simulink model "Australian14gen_R2017a"  (R2017a)
settings: Solver=ode23tb  StartTime=0.0  StopTime=50  FixedStep=1/50  MaxStep=1/50  RelTol=1e-3  AbsTol=1e-1  EnableMultiTasking=on
PreLoadFcn:
  | dataaustralian14gen
values from neighbouring files (symbols this model uses):
  bus_v = [ 101	15 ... (first row only)    [dataaustralian14gen.m]
  comp = [ 1	211	0	0 ... (first row only)    [dataaustralian14gen.m]
  Exc = [ 101	0	 200	0.1	    13.25  2.5	 0	0       0       0       0       0 ... (first row only)    [dataaustralian14gen.m]
  FH = 13    [dataaustralian14gen.m]
  FI = 1    [dataaustralian14gen.m]
  FL = .1    (= 0.1)    [dataaustralian14gen.m]
  G_data = [ 101	333.3	15	3.6	0.14	1.1	0.65	0.25	8.5     0.20	0.05	0       0       0.25	0.2 	0 ... (first row only)    [dataaustralian14gen.m]
  KH = 120    [dataaustralian14gen.m]
  KI = 10    [dataaustralian14gen.m]
  KL = 10    [dataaustralian14gen.m]
  line = [ 102	217	0.0084	0.0667	0.817	330	1 ... (first row only)    [dataaustralian14gen.m]
  p = p_case1    [dataaustralian14gen.m]
  PSSMODEL = 1    [dataaustralian14gen.m]
  SVC = [ 205	650 430   -220 1.055  -68.3 ... (first row only)    [dataaustralian14gen.m]
  trans = [     1   101   102    15   330   333.3    12     12    0.9390 ... (first row only)    [dataaustralian14gen.m]
undefined symbols (not defined in the file or in its folder): D1, Delta
libraries: powerlib x371, sps_avr x14, powerlib_extras x9, factslib x5
(part 3 of 3)

== system Australian14gen_R2017a/NPS_5 ==
  501 : powerlib/Machines/Synchronous Machine pu Standard  PresetModel=No  MechanicalLoad=Mechanical power Pm  ShowDetailedParameters=on  RotorType=Round  Units=per unit standard parameters  MeasurementBus=off  NominalParameters="[G_data(12,2)*1E6  G_data(12,3)*1E3  50]"  Reactances1=[G_data(12,6),G_data(12,8),G_data(12,10),G_data(12,7),G_data(12,12),G_data(12,14),G_data(12,5)]  Reactances2=[G_data(12,6),G_data(12,8),G_data(12,10),G_data(12,7),G_data(12,12),G_data(12,14),G_data(12,5)]  dAxisTimeConstants=Open-circuit  qAxisTimeConstants=Open-circuit  TimeConstants1="[G_data(12,9)  G_data(12,11)  G_data(12,13) G_data(12,15)]"  TimeConstants2="[G_data(12,9)  G_data(12,11)  G_data(12,13) G_data(12,15)]"  TimeConstants3="[  5.9  0.033  0.023  ]"  TimeConstants4=[ 8.0, 0.03, 0.3371, 0.0295 ]  TimeConstants5=[ 1.01, 0.053, 0.1 ]  TimeConstants6=[ 1.3201, 0.023, 1.0, 0.07 ]  TimeConstants7="[  1.01  0.053  0.051266  ]"  TimeConstants8=[ 1.3201, 0.0231, 0.3371, 0.0295 ]  StatorResistance=0  Mechanical="[ G_data(12,4) 0  4 ]"  PolePairs=4  InitialConditions=[0 -93.632 0.904595 0.904595 0.904595 -62.347 -182.347 57.653 2.30263]  SetSaturation=off  Saturation=[0.6404,0.7127,0.8441,0.9214,0.9956,1.082,1.19,1.316,1.457;0.7,0.7698,0.8872,0.9466,0.9969,1.046,1.1,1.151,1.201]  LoadFlowParameters=[1 600000000 20000 0 0]  TsPowergui=0  TsBlock=-1  IterativeModel=Forward Euler  IterativeDiscreteModel=Trapezoidal non iterative  BusType=PV  Pref=p(12,3)*1e6  Qref=0  Qmin=-inf  Qmax=inf  PLF=0  QLF=0
      settings: SourceProductName=Simscape Power Systems
  AC1A Excitation System 501 : sps_avr/AC1A Excitation System  Tr=Exc(12,2)  KaTa="[Exc(12,3)   Exc(12,4)]"  VAminmax=[-14.5 14.5]  VRminmax=[-5.43 6.03]  KfTf="[Exc(12,9)  Exc(12,10)]"  TbTc="[Exc(12,5)  Exc(12,6)]"  KeTe="[Exc(12,7)  Exc(12,8)]"  Ve12=[4.18 3.14]  SeVe12=[0.10 0.03]  Kd=0.38  Kc=0.20  v0=[1 2.3026]  TsBlock=0
      settings: SourceProductName=Simscape Power Systems  SourceProductBaseCode=PS
  Bus Selector1 : BusSelector  OutputSignals="Mechanical.Rotor speed  wm  (pu),Output active power   Peo (pu),Mechanical.Rotor speed deviation  dw (pu),Mechanical.Rotor angle deviation  d_theta (rad),Mechanical.Rotor mechanical angle  theta (deg),dq0 components.Stator voltage  vd (pu),dq0 components.Stator voltage  vq (pu),dq0 components.Field current  ifd (pu),Output reactive power  Qeo (pu)"
  Complex to Magnitude-Angle : ComplexToMagnitudeAngle  Output=Magnitude
  "Delta Pa PSS 501 " : powerlib/Machines/Generic Power System Stabilizer  Tsensor=15e-3  K=2.5*1.25  Twashout=1  Tleadlag1=[60e-3 1]  Tleadlag2=[0 0]  VSlimits=[-0.15 0.15]  Vinit=0  Plot_On=off  MagdB_On=on  FreqRange=logspace(-2,2,500)
      settings: SourceProductName=Simscape Power Systems  SourceProductBaseCode=PS
  "Delta w PSS (Kundur) 501 " : powerlib/Machines/Generic Power System Stabilizer  Tsensor=15e-3  K=30  Twashout=10  Tleadlag1=[50e-3 20e-3]  Tleadlag2=[3 5.4]  VSlimits=[-0.15 0.15]  Vinit=0  Plot_On=off  MagdB_On=on  FreqRange=logspace(-2,2,500)
      settings: SourceProductName=Simscape Power Systems  SourceProductBaseCode=PS
  "MB-PSS 501 " : powerlib/Machines/Multi-Band Power System Stabilizer  OperationMode=Simplified settings  Kg=G  GL="[FL  KL]"  GI="[FI  KI]"  GH="[FH  KH]"  GLd=[66 66 9.4]  TcLF=[1.667 2 0 0 0 0 2 2.4 0 0 0 0 1 1]  GId=[66 66 47.6]  TcIF=[1 1 0.25 0.3 0 0 1 1 0.3 0.36 0 0 0 0]  GHd=[66 66 233]  TcHF="[0.01 0.012 0 0 0 0  0.012 0.0144 0 0 0 0 1 1]"  LIM=[.075 .15 .15 .15]  Plot_On=off  MagdB_On=off  FreqRange=logspace(-2,2,500)
      settings: SourceProductName=Simscape Power Systems  SourceProductBaseCode=PS
  Multiport Switch1 : MultiPortSwitch  Inputs=4  InputSameDT=on
  PSS model3 : Constant  Value=0
  PSS model4 : Constant
  Pref1 : Constant  Value=0.90009
  Real-Imag to Complex : RealImagToComplex
  STG 501 : powerlib/Machines/Steam Turbine and Governor  gentype=Tandem-compound (single mass)  reg1="[ 1  0.05    0 ]"  reg2="[ 0.001  0.15 ]"  reg3="[ -0.1  0.1  0  4.496 ]"  N=3000  turb1="[ 0  10   3.3   0.5   ]"  turb2="[   0   0.36    0.36   0.28   ]"  HA="[ 0.046  1.430  1.465   0.192 ]"  KA="[ 90.44  53.88  64.59   62.94  ]"  DA="[ 0.0115  0.3575  0.3663   0.0137  ]"  ini1=0.90009  ini2=[0.779316,-31.4247]
      settings: SourceProductName=Simscape Power Systems  SourceProductBaseCode=PS
  Scope4 : Scope
  Sum2 : Sum  SaturateOnIntegerOverflow=on  InputSameDT=on  OutDataTypeStr=Inherit: Same as first input
  Sum3 : Sum  Inputs=-+  SaturateOnIntegerOverflow=on  InputSameDT=on  OutDataTypeStr=Inherit: Same as first input
  Vref501 : Constant
  wref : Constant
  A : PMIOPort  Port=1  Side=Left
  B : PMIOPort  Port=2  Side=Left
  C : PMIOPort  Port=3  Side=Left
  tag scope: EFD501=global, Pa501=global, Pe501=global, Pm501=global, Q501=global, Vt501=global, d_theta501=global, pss501=global, theta501=global, w501=global
  wires:
  Bus Selector1/7 -> Real-Imag to Complex/2  "<Stator voltage  vq (pu)>"
  Bus Selector1/6 -> Real-Imag to Complex/1  "<Stator voltage  vd (pu)>"
  wref/1 -> STG 501/1
  Vref501/1 -> AC1A Excitation System 501/1
  Bus Selector1/4 -> STG 501/4, [d_theta501]  "<Rotor angle deviation  d_theta (rad)>"
  501/1 -> [M501], Bus Selector1/1
  Bus Selector1/1 -> [w501], STG 501/3  "<Rotor speed  wm  (pu)>"
  Bus Selector1/3 -> "Delta w PSS (Kundur) 501 "/1, "MB-PSS 501 "/1  "<Rotor speed deviation  dw (pu)>"
  Real-Imag to Complex/1 -> Complex to Magnitude-Angle/1
  Complex to Magnitude-Angle/1 -> AC1A Excitation System 501/2, [Vt501]
  AC1A Excitation System 501/1 -> 501/2, [EFD501]
  Bus Selector1/5 -> [theta501]  "<Rotor mechanical angle  theta (deg)>"
  Bus Selector1/2 -> [Pe501]  "<Output active power   Peo (pu)>"
  Bus Selector1/8 -> AC1A Excitation System 501/3  "<Field current  ifd (pu)>"
  STG 501/4 -> 501/1, [Pm501]
  Bus Selector1/9 -> [Q501]  "<Output reactive power  Qeo (pu)>"
  PSS model4/1 -> Sum2/2
  Sum2/1 -> Multiport Switch1/1
  [PSSmodel] -> Sum2/1
  PSS model3/1 -> Multiport Switch1/2
  Sum3/1 -> [Pa501], "Delta Pa PSS 501 "/1  "Pm-Pe"
  "Delta Pa PSS 501 "/1 -> Multiport Switch1/5
  "Delta w PSS (Kundur) 501 "/1 -> Multiport Switch1/4
  [Pm501] -> Sum3/2
  [Pe501] -> Sum3/1
  "MB-PSS 501 "/1 -> Multiport Switch1/3
  Pref1/1 -> STG 501/2
  Multiport Switch1/1 -> AC1A Excitation System 501/4, Scope4/1, [pss501]
  connections:
  501/RConn1 -- A/RConn1
  501/RConn2 -- B/RConn1
  501/RConn3 -- C/RConn1

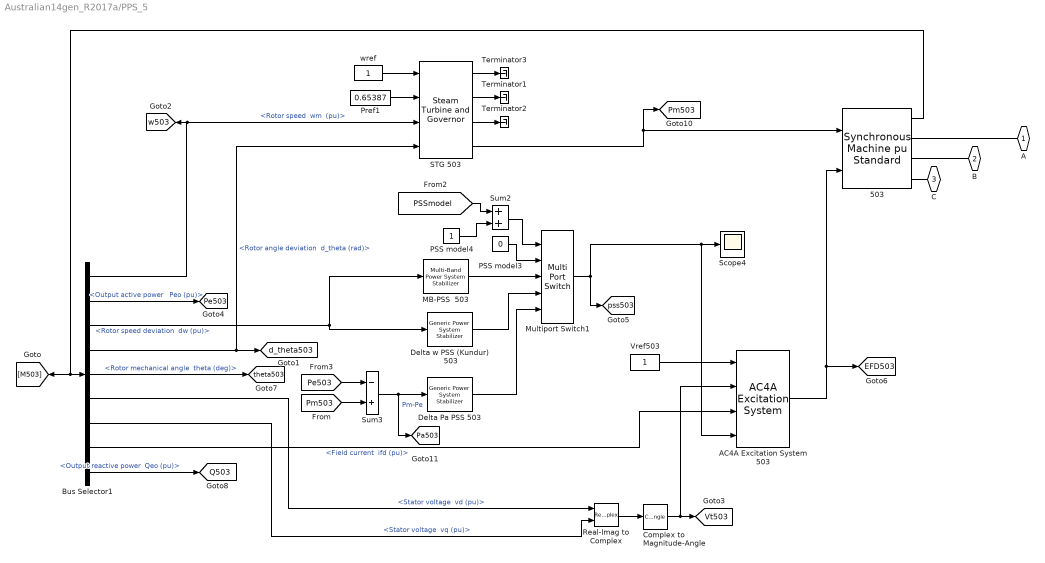
== system Australian14gen_R2017a/PPS_5 ==
  503 : powerlib/Machines/Synchronous Machine pu Standard  PresetModel=No  MechanicalLoad=Mechanical power Pm  ShowDetailedParameters=on  RotorType=Round  Units=per unit standard parameters  MeasurementBus=off  NominalParameters="[G_data(14,2)*1E6  G_data(14,3)*1E3  50]"  Reactances1=[G_data(14,6),G_data(14,8),G_data(14,10),G_data(14,7),G_data(14,12),G_data(14,14),G_data(14,5)]  Reactances2=[G_data(14,6),G_data(14,8),G_data(14,10),G_data(14,7),G_data(14,12),G_data(14,14),G_data(14,5)]  dAxisTimeConstants=Open-circuit  qAxisTimeConstants=Open-circuit  TimeConstants1="[G_data(14,9)  G_data(14,11) G_data(14,13)  G_data(14,15)]"  TimeConstants2="[G_data(14,9)  G_data(14,11) G_data(14,13)  G_data(14,15)]"  TimeConstants3="[  5.9  0.033  0.023  ]"  TimeConstants4=[ 8.0, 0.03, 0.3371, 0.0295 ]  TimeConstants5=[ 1.01, 0.053, 0.1 ]  TimeConstants6=[ 1.3201, 0.023, 1.0, 0.07 ]  TimeConstants7="[  1.01  0.053  0.051266  ]"  TimeConstants8=[ 1.3201, 0.0231, 0.3371, 0.0295 ]  StatorResistance=0  Mechanical=[ G_data(14,4) 0 4 ]  PolePairs=4  InitialConditions=[0 -103.108 0.674862 0.674862 0.674862 -71.8664 -191.866 48.1336 2.0412]  SetSaturation=off  Saturation=[0.6404,0.7127,0.8441,0.9214,0.9956,1.082,1.19,1.316,1.457;0.7,0.7698,0.8872,0.9466,0.9969,1.046,1.1,1.151,1.201]  LoadFlowParameters=[1 436000000 15000 0 0]  TsPowergui=0  TsBlock=-1  IterativeModel=Forward Euler  IterativeDiscreteModel=Trapezoidal non iterative  BusType=PV  Pref=p(14,3)*1e6  Qref=0  Qmin=-inf  Qmax=inf  PLF=0  QLF=0
      settings: SourceProductName=Simscape Power Systems
  AC4A Excitation System 503 : sps_avr/AC4A Excitation System  Tr=Exc(14,2)  KaTa="[Exc(14,3)   Exc(14,4)]"  VIminmax=[-10 10]  VRminmax=[-4.53 5.64]  TbTc="[Exc(14,5)  Exc(14,6)]"  Kc=0  v0=[1 2.0412]  TsBlock=0
      settings: SourceProductName=Simscape Power Systems  SourceProductBaseCode=PS
  Bus Selector1 : BusSelector  OutputSignals="Mechanical.Rotor speed  wm  (pu),Output active power   Peo (pu),Mechanical.Rotor speed deviation  dw (pu),Mechanical.Rotor angle deviation  d_theta (rad),Mechanical.Rotor mechanical angle  theta (deg),dq0 components.Stator voltage  vd (pu),dq0 components.Stator voltage  vq (pu),dq0 components.Field current  ifd (pu),Output reactive power  Qeo (pu)"
  Complex to Magnitude-Angle : ComplexToMagnitudeAngle  Output=Magnitude
  "Delta Pa PSS 503 " : powerlib/Machines/Generic Power System Stabilizer  Tsensor=15e-3  K=2.5*1.25  Twashout=1  Tleadlag1=[60e-3 1]  Tleadlag2=[0 0]  VSlimits=[-0.15 0.15]  Vinit=0  Plot_On=off  MagdB_On=on  FreqRange=logspace(-2,2,500)
      settings: SourceProductName=Simscape Power Systems  SourceProductBaseCode=PS
  Delta w PSS (Kundur)  503 : powerlib/Machines/Generic Power System Stabilizer  Tsensor=15e-3  K=30  Twashout=10  Tleadlag1=[50e-3 20e-3]  Tleadlag2=[3 5.4]  VSlimits=[-0.15 0.15]  Vinit=0  Plot_On=off  MagdB_On=on  FreqRange=logspace(-2,2,500)
      settings: SourceProductName=Simscape Power Systems  SourceProductBaseCode=PS
  MB-PSS  503 : powerlib/Machines/Multi-Band Power System Stabilizer  OperationMode=Simplified settings  Kg=G  GL="[FL  KL]"  GI="[FI  KI]"  GH="[FH  KH]"  GLd=[66 66 9.4]  TcLF=[1.667 2 0 0 0 0 2 2.4 0 0 0 0 1 1]  GId=[66 66 47.6]  TcIF=[1 1 0.25 0.3 0 0 1 1 0.3 0.36 0 0 0 0]  GHd=[66 66 233]  TcHF="[0.01 0.012 0 0 0 0  0.012 0.0144 0 0 0 0 1 1]"  LIM=[.075 .15 .15 .15]  Plot_On=off  MagdB_On=off  FreqRange=logspace(-2,2,500)
      settings: SourceProductName=Simscape Power Systems  SourceProductBaseCode=PS
  Multiport Switch1 : MultiPortSwitch  Inputs=4  InputSameDT=on
  PSS model3 : Constant  Value=0
  PSS model4 : Constant
  Pref1 : Constant  Value=0.65387
  Real-Imag to Complex : RealImagToComplex
  STG 503 : powerlib/Machines/Steam Turbine and Governor  gentype=Tandem-compound (single mass)  reg1="[ 1  0.05    0 ]"  reg2="[ 0.001  0.15 ]"  reg3="[ -0.1  0.1  0  4.496 ]"  N=3000  turb1="[ 0  10   3.3   0.5   ]"  turb2="[   0   0.36    0.36   0.28   ]"  HA="[ 0.046  1.430  1.465   0.192 ]"  KA="[ 90.44  53.88  64.59   62.94  ]"  DA="[ 0.0115  0.3575  0.3663   0.0137  ]"  ini1=0.65387  ini2=[0.779316,-31.4247]
      settings: SourceProductName=Simscape Power Systems  SourceProductBaseCode=PS
  Scope4 : Scope
  Sum2 : Sum  SaturateOnIntegerOverflow=on  InputSameDT=on  OutDataTypeStr=Inherit: Same as first input
  Sum3 : Sum  Inputs=-+  SaturateOnIntegerOverflow=on  InputSameDT=on  OutDataTypeStr=Inherit: Same as first input
  Terminator1 : Terminator
  Terminator2 : Terminator
  Terminator3 : Terminator
  Vref503 : Constant
  wref : Constant
  A : PMIOPort  Port=1  Side=Left
  B : PMIOPort  Port=2  Side=Left
  C : PMIOPort  Port=3  Side=Left
  tag scope: EFD503=global, Pa503=global, Pe503=global, Pm503=global, Q503=global, Vt503=global, d_theta503=global, pss503=global, theta503=global, w503=global
  wires:
  Bus Selector1/7 -> Real-Imag to Complex/2  "<Stator voltage  vq (pu)>"
  Bus Selector1/6 -> Real-Imag to Complex/1  "<Stator voltage  vd (pu)>"
  wref/1 -> STG 503/1
  Vref503/1 -> AC4A Excitation System 503/1
  Bus Selector1/4 -> STG 503/4, [d_theta503]  "<Rotor angle deviation  d_theta (rad)>"
  503/1 -> [M503], Bus Selector1/1
  Bus Selector1/1 -> [w503], STG 503/3  "<Rotor speed  wm  (pu)>"
  Bus Selector1/3 -> MB-PSS  503/1, Delta w PSS (Kundur)  503/1  "<Rotor speed deviation  dw (pu)>"
  Real-Imag to Complex/1 -> Complex to Magnitude-Angle/1
  Complex to Magnitude-Angle/1 -> AC4A Excitation System 503/2, [Vt503]
  AC4A Excitation System 503/1 -> 503/2, [EFD503]
  Bus Selector1/5 -> [theta503]  "<Rotor mechanical angle  theta (deg)>"
  Bus Selector1/2 -> [Pe503]  "<Output active power   Peo (pu)>"
  Bus Selector1/8 -> AC4A Excitation System 503/3  "<Field current  ifd (pu)>"
  STG 503/4 -> 503/1, [Pm503]
  Bus Selector1/9 -> [Q503]  "<Output reactive power  Qeo (pu)>"
  PSS model4/1 -> Sum2/2
  Sum2/1 -> Multiport Switch1/1
  [PSSmodel] -> Sum2/1
  PSS model3/1 -> Multiport Switch1/2
  Sum3/1 -> [Pa503], "Delta Pa PSS 503 "/1  "Pm-Pe"
  "Delta Pa PSS 503 "/1 -> Multiport Switch1/5
  Delta w PSS (Kundur)  503/1 -> Multiport Switch1/4
  [Pm503] -> Sum3/2
  [Pe503] -> Sum3/1
  MB-PSS  503/1 -> Multiport Switch1/3
  STG 503/1 -> Terminator3/1
  STG 503/2 -> Terminator1/1
  STG 503/3 -> Terminator2/1
  Pref1/1 -> STG 503/2
  Multiport Switch1/1 -> AC4A Excitation System 503/4, Scope4/1, [pss503]
  connections:
  503/RConn1 -- A/RConn1
  503/RConn2 -- B/RConn1
  503/RConn3 -- C/RConn1

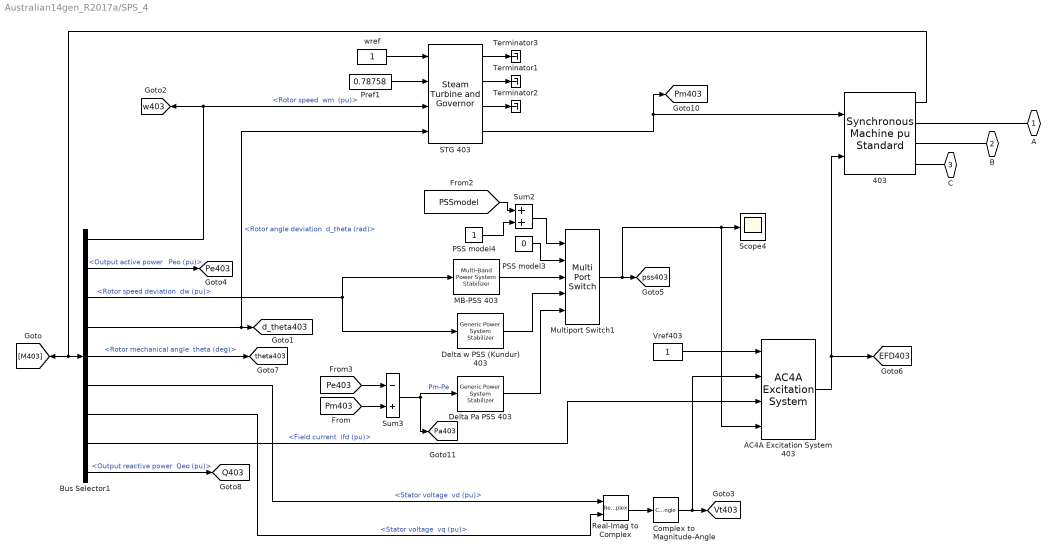
== system Australian14gen_R2017a/SPS_4 ==
  403 : powerlib/Machines/Synchronous Machine pu Standard  PresetModel=No  MechanicalLoad=Mechanical power Pm  ShowDetailedParameters=on  RotorType=Round  Units=per unit standard parameters  MeasurementBus=off  NominalParameters="[G_data(10,2)*1E6  G_data(10,3)*1E3  50]"  Reactances1=[G_data(10,6),G_data(10,8),G_data(10,10),G_data(10,7),G_data(10,12),G_data(10,14),G_data(10,5)]  Reactances2=[G_data(10,6),G_data(10,8),G_data(10,10),G_data(10,7),G_data(10,12),G_data(10,14),G_data(10,5)]  dAxisTimeConstants=Open-circuit  qAxisTimeConstants=Open-circuit  TimeConstants1="[G_data(10,9)  G_data(10,11)  G_data(10,13)  G_data(10,15)]"  TimeConstants2="[G_data(10,9)  G_data(10,11)  G_data(10,13)  G_data(10,15)]"  TimeConstants3="[  5.9  0.033  0.023  ]"  TimeConstants4=[ 8.0, 0.03, 0.3371, 0.0295 ]  TimeConstants5=[ 1.01, 0.053, 0.1 ]  TimeConstants6=[ 1.3201, 0.023, 1.0, 0.07 ]  TimeConstants7="[  1.01  0.053  0.051266  ]"  TimeConstants8=[ 1.3201, 0.0231, 0.3371, 0.0295 ]  StatorResistance=0  Mechanical="[ G_data(10,4) 0  4 ]"  PolePairs=4  InitialConditions=[0 67.1142 0.796278 0.796278 0.796278 100.495 -19.5047 220.495 2.1966]  SetSaturation=off  Saturation=[0.6404,0.7127,0.8441,0.9214,0.9956,1.082,1.19,1.316,1.457;0.7,0.7698,0.8872,0.9466,0.9969,1.046,1.1,1.151,1.201]  LoadFlowParameters=[1 1400000000 20000 0 0]  TsPowergui=0  TsBlock=-1  IterativeModel=Forward Euler  IterativeDiscreteModel=Trapezoidal non iterative  BusType=PV  Pref=p(10,3)*1e6  Qref=0  Qmin=-inf  Qmax=inf  PLF=0  QLF=0
      settings: SourceProductName=Simscape Power Systems
  AC4A Excitation System 403 : sps_avr/AC4A Excitation System  Tr=Exc(10,2)  KaTa="[Exc(10,3)   Exc(10,4)]"  VIminmax=[-10 10]  VRminmax=[-4.53 5.64]  TbTc="[Exc(10,5)  Exc(10,6)]"  Kc=0  v0=[1 2.1966]  TsBlock=0
      settings: SourceProductName=Simscape Power Systems  SourceProductBaseCode=PS
  Bus Selector1 : BusSelector  OutputSignals="Mechanical.Rotor speed  wm  (pu),Output active power   Peo (pu),Mechanical.Rotor speed deviation  dw (pu),Mechanical.Rotor angle deviation  d_theta (rad),Mechanical.Rotor mechanical angle  theta (deg),dq0 components.Stator voltage  vd (pu),dq0 components.Stator voltage  vq (pu),dq0 components.Field current  ifd (pu),Output reactive power  Qeo (pu)"
  Complex to Magnitude-Angle : ComplexToMagnitudeAngle  Output=Magnitude
  "Delta Pa PSS 403 " : powerlib/Machines/Generic Power System Stabilizer  Tsensor=15e-3  K=2.5*1.25  Twashout=1  Tleadlag1=[60e-3 1]  Tleadlag2=[0 0]  VSlimits=[-0.15 0.15]  Vinit=0  Plot_On=off  MagdB_On=on  FreqRange=logspace(-2,2,500)
      settings: SourceProductName=Simscape Power Systems  SourceProductBaseCode=PS
  Delta w PSS (Kundur) 403 : powerlib/Machines/Generic Power System Stabilizer  Tsensor=15e-3  K=30  Twashout=10  Tleadlag1=[50e-3 20e-3]  Tleadlag2=[3 5.4]  VSlimits=[-0.15 0.15]  Vinit=0  Plot_On=off  MagdB_On=on  FreqRange=logspace(-2,2,500)
      settings: SourceProductName=Simscape Power Systems  SourceProductBaseCode=PS
  "MB-PSS 403 " : powerlib/Machines/Multi-Band Power System Stabilizer  OperationMode=Simplified settings  Kg=G  GL="[FL  KL]"  GI="[FI  KI]"  GH="[FH  KH]"  GLd=[66 66 9.4]  TcLF=[1.667 2 0 0 0 0 2 2.4 0 0 0 0 1 1]  GId=[66 66 47.6]  TcIF=[1 1 0.25 0.3 0 0 1 1 0.3 0.36 0 0 0 0]  GHd=[66 66 233]  TcHF="[0.01 0.012 0 0 0 0  0.012 0.0144 0 0 0 0 1 1]"  LIM=[.075 .15 .15 .15]  Plot_On=off  MagdB_On=off  FreqRange=logspace(-2,2,500)
      settings: SourceProductName=Simscape Power Systems  SourceProductBaseCode=PS
  Multiport Switch1 : MultiPortSwitch  Inputs=4  InputSameDT=on
  PSS model3 : Constant  Value=0
  PSS model4 : Constant
  Pref1 : Constant  Value=0.78758
  Real-Imag to Complex : RealImagToComplex
  STG 403 : powerlib/Machines/Steam Turbine and Governor  gentype=Tandem-compound (single mass)  reg1="[ 1  0.05    0 ]"  reg2="[ 0.001  0.15 ]"  reg3="[ -0.1  0.1  0  4.496 ]"  N=3000  turb1="[ 0  10   3.3   0.5   ]"  turb2="[   0   0.36    0.36   0.28   ]"  HA="[ 0.046  1.430  1.465   0.192 ]"  KA="[ 90.44  53.88  64.59   62.94  ]"  DA="[ 0.0115  0.3575  0.3663   0.0137  ]"  ini1=0.78758  ini2=[0.779316,-31.4247]
      settings: SourceProductName=Simscape Power Systems  SourceProductBaseCode=PS
  Scope4 : Scope
  Sum2 : Sum  SaturateOnIntegerOverflow=on  InputSameDT=on  OutDataTypeStr=Inherit: Same as first input
  Sum3 : Sum  Inputs=-+  SaturateOnIntegerOverflow=on  InputSameDT=on  OutDataTypeStr=Inherit: Same as first input
  Terminator1 : Terminator
  Terminator2 : Terminator
  Terminator3 : Terminator
  Vref403 : Constant
  wref : Constant
  A : PMIOPort  Port=1  Side=Left
  B : PMIOPort  Port=2  Side=Left
  C : PMIOPort  Port=3  Side=Left
  tag scope: EFD403=global, Pa403=global, Pe403=global, Pm403=global, Q403=global, Vt403=global, d_theta403=global, pss403=global, theta403=global, w403=global
  wires:
  Bus Selector1/7 -> Real-Imag to Complex/2  "<Stator voltage  vq (pu)>"
  Bus Selector1/6 -> Real-Imag to Complex/1  "<Stator voltage  vd (pu)>"
  wref/1 -> STG 403/1
  Vref403/1 -> AC4A Excitation System 403/1
  Bus Selector1/4 -> STG 403/4, [d_theta403]  "<Rotor angle deviation  d_theta (rad)>"
  403/1 -> [M403], Bus Selector1/1
  Bus Selector1/1 -> [w403], STG 403/3  "<Rotor speed  wm  (pu)>"
  Bus Selector1/3 -> Delta w PSS (Kundur) 403/1, "MB-PSS 403 "/1  "<Rotor speed deviation  dw (pu)>"
  Real-Imag to Complex/1 -> Complex to Magnitude-Angle/1
  Complex to Magnitude-Angle/1 -> AC4A Excitation System 403/2, [Vt403]
  AC4A Excitation System 403/1 -> 403/2, [EFD403]
  Bus Selector1/5 -> [theta403]  "<Rotor mechanical angle  theta (deg)>"
  Bus Selector1/2 -> [Pe403]  "<Output active power   Peo (pu)>"
  Bus Selector1/8 -> AC4A Excitation System 403/3  "<Field current  ifd (pu)>"
  STG 403/4 -> 403/1, [Pm403]
  Bus Selector1/9 -> [Q403]  "<Output reactive power  Qeo (pu)>"
  PSS model4/1 -> Sum2/2
  Sum2/1 -> Multiport Switch1/1
  [PSSmodel] -> Sum2/1
  PSS model3/1 -> Multiport Switch1/2
  Sum3/1 -> [Pa403], "Delta Pa PSS 403 "/1  "Pm-Pe"
  "Delta Pa PSS 403 "/1 -> Multiport Switch1/5
  Delta w PSS (Kundur) 403/1 -> Multiport Switch1/4
  [Pm403] -> Sum3/2
  [Pe403] -> Sum3/1
  "MB-PSS 403 "/1 -> Multiport Switch1/3
  STG 403/1 -> Terminator3/1
  STG 403/2 -> Terminator1/1
  STG 403/3 -> Terminator2/1
  Pref1/1 -> STG 403/2
  Multiport Switch1/1 -> AC4A Excitation System 403/4, Scope4/1, [pss403]
  connections:
  403/RConn1 -- A/RConn1
  403/RConn2 -- B/RConn1
  403/RConn3 -- C/RConn1

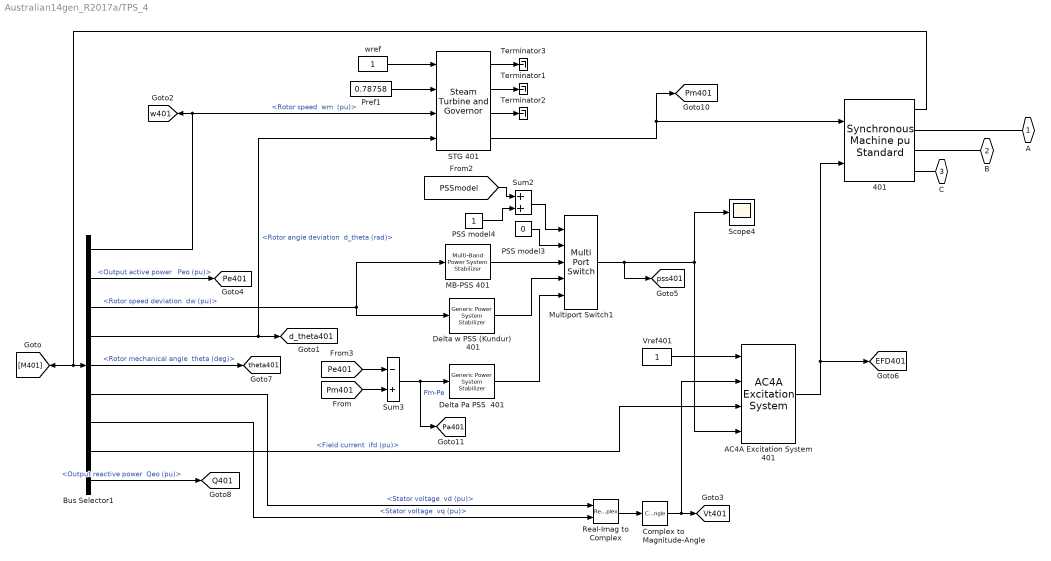
== system Australian14gen_R2017a/TPS_4 ==
  401 : powerlib/Machines/Synchronous Machine pu Standard  PresetModel=No  MechanicalLoad=Mechanical power Pm  ShowDetailedParameters=on  RotorType=Round  Units=per unit standard parameters  MeasurementBus=off  NominalParameters="[G_data(8,2)*1E6  G_data(8,3)*1E3  50]"  Reactances1=[G_data(8,6),G_data(8,8),G_data(8,10),G_data(8,7),G_data(8,12),G_data(8,14),G_data(8,5)]  Reactances2=[G_data(8,6),G_data(8,8),G_data(8,10),G_data(8,7),G_data(8,14),G_data(8,5)]  dAxisTimeConstants=Open-circuit  qAxisTimeConstants=Open-circuit  TimeConstants1="[G_data(8,9)  G_data(8,11)  G_data(8,15)]"  TimeConstants2="[G_data(8,9)  G_data(8,11)  G_data(8,13)  G_data(8,15)]"  TimeConstants3="[  5.9  0.033  0.023  ]"  TimeConstants4=[ 8.0, 0.03, 0.3371, 0.0295 ]  TimeConstants5=[ 1.01, 0.053, 0.1 ]  TimeConstants6=[ 1.3201, 0.023, 1.0, 0.07 ]  TimeConstants7="[  1.01  0.053  0.051266  ]"  TimeConstants8=[ 1.3201, 0.0231, 0.3371, 0.0295 ]  StatorResistance=0  Mechanical="[ G_data(8,4) 0  4 ]"  PolePairs=4  InitialConditions=[0 23.0374 0.837012 0.837012 0.837012 51.1473 -68.8527 171.147 2.44002]  SetSaturation=off  Saturation=[0.6404,0.7127,0.8441,0.9214,0.9956,1.082,1.19,1.316,1.457;0.7,0.7698,0.8872,0.9466,0.9969,1.046,1.1,1.151,1.201]  LoadFlowParameters=[1 1400000000 20000 0 0]  TsPowergui=0  TsBlock=-1  IterativeModel=Forward Euler  IterativeDiscreteModel=Trapezoidal non iterative  BusType=PV  Pref=p(8,3)*1e6  Qref=0  Qmin=-inf  Qmax=inf  PLF=0  QLF=0
      settings: SourceProductName=Simscape Power Systems
  AC4A Excitation System 401 : sps_avr/AC4A Excitation System  Tr=Exc(8,2)  KaTa="[Exc(8,3)   Exc(8,4)]"  VIminmax=[-10 10]  VRminmax=[-4.53 5.64]  TbTc="[Exc(8,5)  Exc(8,6)]"  Kc=0  v0=[1 2.44]  TsBlock=0
      settings: SourceProductName=Simscape Power Systems  SourceProductBaseCode=PS
  Bus Selector1 : BusSelector  OutputSignals="Mechanical.Rotor speed  wm  (pu),Output active power   Peo (pu),Mechanical.Rotor speed deviation  dw (pu),Mechanical.Rotor angle deviation  d_theta (rad),Mechanical.Rotor mechanical angle  theta (deg),dq0 components.Stator voltage  vd (pu),dq0 components.Stator voltage  vq (pu),dq0 components.Field current  ifd (pu),Output reactive power  Qeo (pu)"
  Complex to Magnitude-Angle : ComplexToMagnitudeAngle  Output=Magnitude
  Delta Pa PSS  401 : powerlib/Machines/Generic Power System Stabilizer  Tsensor=15e-3  K=2.5*1.25  Twashout=1  Tleadlag1=[60e-3 1]  Tleadlag2=[0 0]  VSlimits=[-0.15 0.15]  Vinit=0  Plot_On=off  MagdB_On=on  FreqRange=logspace(-2,2,500)
      settings: SourceProductName=Simscape Power Systems  SourceProductBaseCode=PS
  Delta w PSS (Kundur)  401 : powerlib/Machines/Generic Power System Stabilizer  Tsensor=15e-3  K=30  Twashout=10  Tleadlag1=[50e-3 20e-3]  Tleadlag2=[3 5.4]  VSlimits=[-0.15 0.15]  Vinit=0  Plot_On=off  MagdB_On=on  FreqRange=logspace(-2,2,500)
      settings: SourceProductName=Simscape Power Systems  SourceProductBaseCode=PS
  "MB-PSS 401 " : powerlib/Machines/Multi-Band Power System Stabilizer  OperationMode=Simplified settings  Kg=G  GL="[FL  KL]"  GI="[FI  KI]"  GH="[FH  KH]"  GLd=[66 66 9.4]  TcLF=[1.667 2 0 0 0 0 2 2.4 0 0 0 0 1 1]  GId=[66 66 47.6]  TcIF=[1 1 0.25 0.3 0 0 1 1 0.3 0.36 0 0 0 0]  GHd=[66 66 233]  TcHF="[0.01 0.012 0 0 0 0  0.012 0.0144 0 0 0 0 1 1]"  LIM=[.075 .15 .15 .15]  Plot_On=off  MagdB_On=off  FreqRange=logspace(-2,2,500)
      settings: SourceProductName=Simscape Power Systems  SourceProductBaseCode=PS
  Multiport Switch1 : MultiPortSwitch  Inputs=4  InputSameDT=on
  PSS model3 : Constant  Value=0
  PSS model4 : Constant
  Pref1 : Constant  Value=0.78758
  Real-Imag to Complex : RealImagToComplex
  STG 401 : powerlib/Machines/Steam Turbine and Governor  gentype=Tandem-compound (single mass)  reg1="[ 1  0.05    0 ]"  reg2="[ 0.001  0.15 ]"  reg3="[ -0.1  0.1  0  4.496 ]"  N=3000  turb1="[ 0  10   3.3   0.5   ]"  turb2="[   0   0.36    0.36   0.28   ]"  HA="[ 0.046  1.430  1.465   0.192 ]"  KA="[ 90.44  53.88  64.59   62.94  ]"  DA="[ 0.0115  0.3575  0.3663   0.0137  ]"  ini1=0.78758  ini2=[0.779316,-31.4247]
      settings: SourceProductName=Simscape Power Systems  SourceProductBaseCode=PS
  Scope4 : Scope
  Sum2 : Sum  SaturateOnIntegerOverflow=on  InputSameDT=on  OutDataTypeStr=Inherit: Same as first input
  Sum3 : Sum  Inputs=-+  SaturateOnIntegerOverflow=on  InputSameDT=on  OutDataTypeStr=Inherit: Same as first input
  Terminator1 : Terminator
  Terminator2 : Terminator
  Terminator3 : Terminator
  Vref401 : Constant
  wref : Constant
  A : PMIOPort  Port=1  Side=Left
  B : PMIOPort  Port=2  Side=Left
  C : PMIOPort  Port=3  Side=Left
  tag scope: EFD401=global, Pa401=global, Pe401=global, Pm401=global, Q401=global, Vt401=global, d_theta401=global, pss401=global, theta401=global, w401=global
  wires:
  Bus Selector1/7 -> Real-Imag to Complex/2  "<Stator voltage  vq (pu)>"
  Bus Selector1/6 -> Real-Imag to Complex/1  "<Stator voltage  vd (pu)>"
  wref/1 -> STG 401/1
  Vref401/1 -> AC4A Excitation System 401/1
  Bus Selector1/4 -> STG 401/4, [d_theta401]  "<Rotor angle deviation  d_theta (rad)>"
  401/1 -> [M401], Bus Selector1/1
  Bus Selector1/1 -> [w401], STG 401/3  "<Rotor speed  wm  (pu)>"
  Bus Selector1/3 -> Delta w PSS (Kundur)  401/1, "MB-PSS 401 "/1  "<Rotor speed deviation  dw (pu)>"
  Real-Imag to Complex/1 -> Complex to Magnitude-Angle/1
  Complex to Magnitude-Angle/1 -> AC4A Excitation System 401/2, [Vt401]
  AC4A Excitation System 401/1 -> 401/2, [EFD401]
  Bus Selector1/5 -> [theta401]  "<Rotor mechanical angle  theta (deg)>"
  Bus Selector1/2 -> [Pe401]  "<Output active power   Peo (pu)>"
  Bus Selector1/8 -> AC4A Excitation System 401/3  "<Field current  ifd (pu)>"
  STG 401/4 -> 401/1, [Pm401]
  Bus Selector1/9 -> [Q401]  "<Output reactive power  Qeo (pu)>"
  PSS model4/1 -> Sum2/2
  Sum2/1 -> Multiport Switch1/1
  [PSSmodel] -> Sum2/1
  PSS model3/1 -> Multiport Switch1/2
  Sum3/1 -> [Pa401], Delta Pa PSS  401/1  "Pm-Pe"
  Delta Pa PSS  401/1 -> Multiport Switch1/5
  Delta w PSS (Kundur)  401/1 -> Multiport Switch1/4
  [Pm401] -> Sum3/2
  [Pe401] -> Sum3/1
  "MB-PSS 401 "/1 -> Multiport Switch1/3
  STG 401/1 -> Terminator3/1
  STG 401/2 -> Terminator1/1
  STG 401/3 -> Terminator2/1
  Pref1/1 -> STG 401/2
  Multiport Switch1/1 -> Scope4/1, AC4A Excitation System 401/4, [pss401]
  connections:
  401/RConn1 -- A/RConn1
  401/RConn2 -- B/RConn1
  401/RConn3 -- C/RConn1

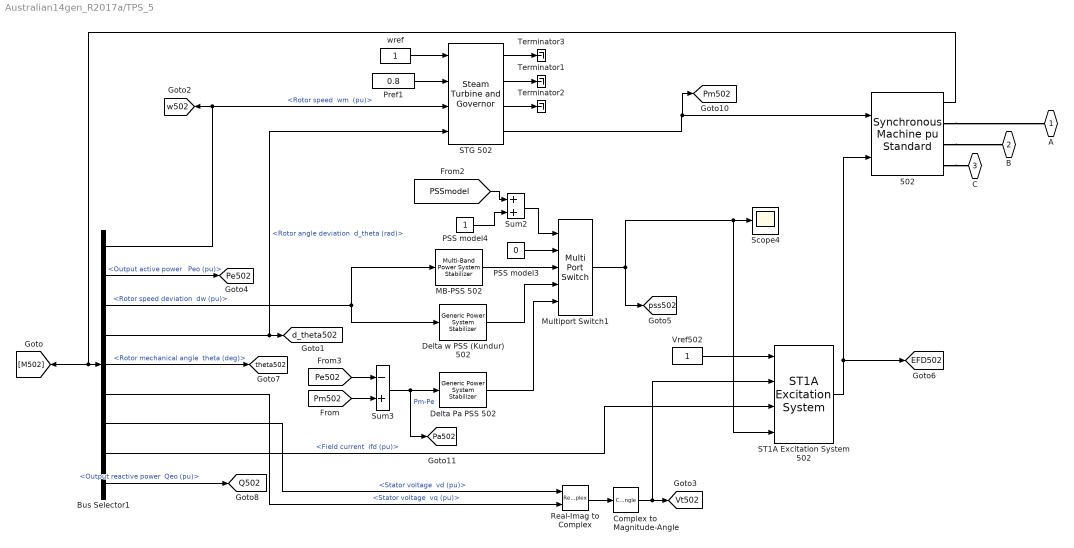
== system Australian14gen_R2017a/TPS_5 ==
  502 : powerlib/Machines/Synchronous Machine pu Standard  PresetModel=No  MechanicalLoad=Mechanical power Pm  ShowDetailedParameters=on  RotorType=Round  Units=per unit standard parameters  MeasurementBus=off  NominalParameters="[G_data(13,2)*1E6  G_data(13,3)*1E3  50]"  Reactances1=[G_data(13,6),G_data(13,8),G_data(13,10),G_data(13,7),G_data(13,12),G_data(13,14),G_data(13,5)]  Reactances2=[G_data(13,6),G_data(13,8),G_data(13,10),G_data(13,7),G_data(13,14),G_data(13,5)]  dAxisTimeConstants=Open-circuit  qAxisTimeConstants=Open-circuit  TimeConstants1="[G_data(13,9)  G_data(13,11)  G_data(13,15)]"  TimeConstants2="[G_data(13,9)  G_data(13,11)  G_data(13,13)  G_data(13,15)]"  TimeConstants3="[  5.9  0.033  0.023  ]"  TimeConstants4=[ 8.0, 0.03, 0.3371, 0.0295 ]  TimeConstants5=[ 1.01, 0.053, 0.1 ]  TimeConstants6=[ 1.3201, 0.023, 1.0, 0.07 ]  TimeConstants7="[  1.01  0.053  0.051266  ]"  TimeConstants8=[ 1.3201, 0.0231, 0.3371, 0.0295 ]  StatorResistance=0  Mechanical="[ G_data(13,4) 0  4 ]"  PolePairs=4  InitialConditions=[0 -101.676 0.818957 0.818957 0.818957 -67.5672 -187.567 52.4328 2.08105]  SetSaturation=off  Saturation=[0.6404,0.7127,0.8441,0.9214,0.9956,1.082,1.19,1.316,1.457;0.7,0.7698,0.8872,0.9466,0.9969,1.046,1.1,1.151,1.201]  LoadFlowParameters=[1 800000000 15000 0 0]  TsPowergui=0  TsBlock=-1  IterativeModel=Forward Euler  IterativeDiscreteModel=Trapezoidal non iterative  BusType=PV  Pref=p(13,3)*1e6  Qref=0  Qmin=-inf  Qmax=inf  PLF=0  QLF=0
      settings: SourceProductName=Simscape Power Systems
  Bus Selector1 : BusSelector  OutputSignals="Mechanical.Rotor speed  wm  (pu),Output active power   Peo (pu),Mechanical.Rotor speed deviation  dw (pu),Mechanical.Rotor angle deviation  d_theta (rad),Mechanical.Rotor mechanical angle  theta (deg),dq0 components.Stator voltage  vq (pu),dq0 components.Stator voltage  vd (pu),dq0 components.Field current  ifd (pu),Output reactive power  Qeo (pu)"
  Complex to Magnitude-Angle : ComplexToMagnitudeAngle  Output=Magnitude
  "Delta Pa PSS 502 " : powerlib/Machines/Generic Power System Stabilizer  Tsensor=15e-3  K=2.5*1.25  Twashout=1  Tleadlag1=[60e-3 1]  Tleadlag2=[0 0]  VSlimits=[-0.15 0.15]  Vinit=0  Plot_On=off  MagdB_On=on  FreqRange=logspace(-2,2,500)
      settings: SourceProductName=Simscape Power Systems  SourceProductBaseCode=PS
  Delta w PSS (Kundur) 502 : powerlib/Machines/Generic Power System Stabilizer  Tsensor=15e-3  K=30  Twashout=10  Tleadlag1=[50e-3 20e-3]  Tleadlag2=[3 5.4]  VSlimits=[-0.15 0.15]  Vinit=0  Plot_On=off  MagdB_On=on  FreqRange=logspace(-2,2,500)
      settings: SourceProductName=Simscape Power Systems  SourceProductBaseCode=PS
  "MB-PSS 502 " : powerlib/Machines/Multi-Band Power System Stabilizer  OperationMode=Simplified settings  Kg=G  GL="[FL  KL]"  GI="[FI  KI]"  GH="[FH  KH]"  GLd=[66 66 9.4]  TcLF=[1.667 2 0 0 0 0 2 2.4 0 0 0 0 1 1]  GId=[66 66 47.6]  TcIF=[1 1 0.25 0.3 0 0 1 1 0.3 0.36 0 0 0 0]  GHd=[66 66 233]  TcHF="[0.01 0.012 0 0 0 0  0.012 0.0144 0 0 0 0 1 1]"  LIM=[.075 .15 .15 .15]  Plot_On=off  MagdB_On=off  FreqRange=logspace(-2,2,500)
      settings: SourceProductName=Simscape Power Systems  SourceProductBaseCode=PS
  Multiport Switch1 : MultiPortSwitch  Inputs=4  InputSameDT=on
  PSS model3 : Constant  Value=0
  PSS model4 : Constant
  Pref1 : Constant  Value=0.8
  Real-Imag to Complex : RealImagToComplex
  ST1A Excitation System 502 : sps_avr/ST1A Excitation System  Tr=Exc(13,2)  KaTa="[Exc(13,3)   Exc(13,4)]"  VIminmax=[-999 +999]  VAminmax=[-999 999]  VRminmax=[-6.0 6.43]  KfTf="[Exc(13,9)  Exc(13,10)]"  TbTc="[Exc(13,5)  Exc(13,6) Exc(13,11)  Exc(13,12)]"  KLR=1  ILR=2  Kc=0.038  v0=[1 2.0811]  TsBlock=0
      settings: SourceProductName=Simscape Power Systems  SourceProductBaseCode=PS
  STG 502 : powerlib/Machines/Steam Turbine and Governor  gentype=Tandem-compound (single mass)  reg1="[ 1  0.05    0 ]"  reg2="[ 0.001  0.15 ]"  reg3="[ -0.1  0.1  0  4.496 ]"  N=3000  turb1="[ 0  10   3.3   0.5   ]"  turb2="[   0   0.36    0.36   0.28   ]"  HA="[ 0.046  1.430  1.465   0.192 ]"  KA="[ 90.44  53.88  64.59   62.94  ]"  DA="[ 0.0115  0.3575  0.3663   0.0137  ]"  ini1=0.8  ini2=[0.779316,-31.4247]
      settings: SourceProductName=Simscape Power Systems  SourceProductBaseCode=PS
  Scope4 : Scope
  Sum2 : Sum  SaturateOnIntegerOverflow=on  InputSameDT=on  OutDataTypeStr=Inherit: Same as first input
  Sum3 : Sum  Inputs=-+  SaturateOnIntegerOverflow=on  InputSameDT=on  OutDataTypeStr=Inherit: Same as first input
  Terminator1 : Terminator
  Terminator2 : Terminator
  Terminator3 : Terminator
  Vref502 : Constant
  wref : Constant
  A : PMIOPort  Port=1  Side=Left
  B : PMIOPort  Port=2  Side=Left
  C : PMIOPort  Port=3  Side=Left
  tag scope: EFD502=global, Pa502=global, Pe502=global, Pm502=global, Q502=global, Vt502=global, d_theta502=global, pss502=global, theta502=global, w502=global
  wires:
  Bus Selector1/6 -> Real-Imag to Complex/2  "<Stator voltage  vq (pu)>"
  Bus Selector1/7 -> Real-Imag to Complex/1  "<Stator voltage  vd (pu)>"
  wref/1 -> STG 502/1
  Vref502/1 -> ST1A Excitation System 502/1
  Bus Selector1/4 -> STG 502/4, [d_theta502]  "<Rotor angle deviation  d_theta (rad)>"
  502/1 -> Bus Selector1/1, [M502]
  Bus Selector1/1 -> [w502], STG 502/3  "<Rotor speed  wm  (pu)>"
  Bus Selector1/3 -> Delta w PSS (Kundur) 502/1, "MB-PSS 502 "/1  "<Rotor speed deviation  dw (pu)>"
  Real-Imag to Complex/1 -> Complex to Magnitude-Angle/1
  Complex to Magnitude-Angle/1 -> ST1A Excitation System 502/2, [Vt502]
  ST1A Excitation System 502/1 -> 502/2, [EFD502]
  Bus Selector1/5 -> [theta502]  "<Rotor mechanical angle  theta (deg)>"
  Bus Selector1/2 -> [Pe502]  "<Output active power   Peo (pu)>"
  Bus Selector1/8 -> ST1A Excitation System 502/3  "<Field current  ifd (pu)>"
  STG 502/4 -> 502/1, [Pm502]
  Bus Selector1/9 -> [Q502]  "<Output reactive power  Qeo (pu)>"
  PSS model4/1 -> Sum2/2
  Sum2/1 -> Multiport Switch1/1
  [PSSmodel] -> Sum2/1
  PSS model3/1 -> Multiport Switch1/2
  Sum3/1 -> [Pa502], "Delta Pa PSS 502 "/1  "Pm-Pe"
  "Delta Pa PSS 502 "/1 -> Multiport Switch1/5
  Delta w PSS (Kundur) 502/1 -> Multiport Switch1/4
  [Pm502] -> Sum3/2
  [Pe502] -> Sum3/1
  "MB-PSS 502 "/1 -> Multiport Switch1/3
  STG 502/1 -> Terminator3/1
  STG 502/2 -> Terminator1/1
  STG 502/3 -> Terminator2/1
  Pref1/1 -> STG 502/2
  Multiport Switch1/1 -> ST1A Excitation System 502/4, Scope4/1, [pss502]
  connections:
  502/RConn1 -- A/RConn1
  502/RConn2 -- B/RConn1
  502/RConn3 -- C/RConn1

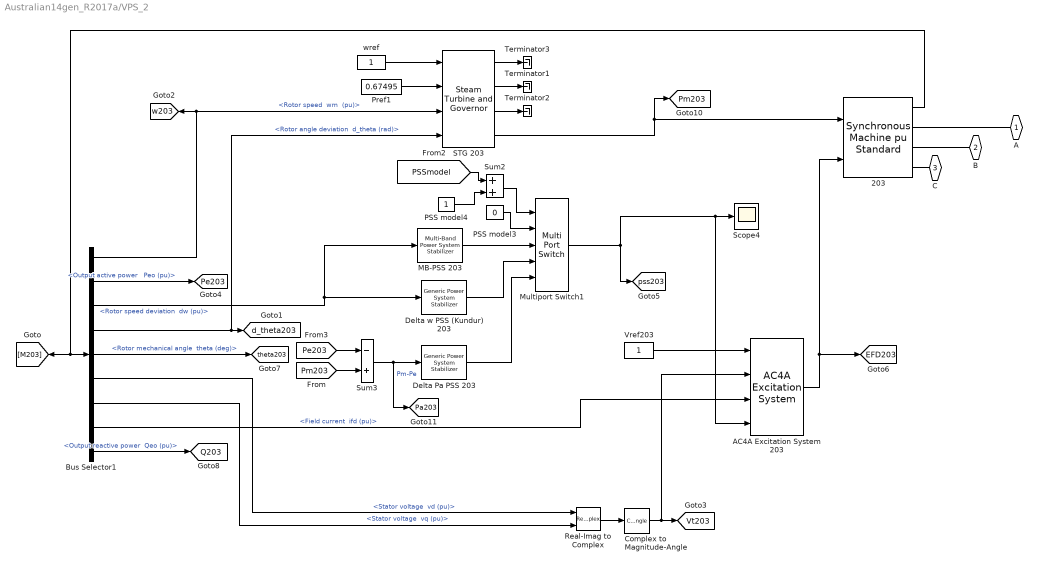
== system Australian14gen_R2017a/VPS_2 ==
  203 : powerlib/Machines/Synchronous Machine pu Standard  PresetModel=No  MechanicalLoad=Mechanical power Pm  ShowDetailedParameters=on  RotorType=Round  Units=per unit standard parameters  MeasurementBus=off  NominalParameters="[G_data(4,2)*1E6  G_data(4,3)*1E3  50]"  Reactances1=[G_data(4,6),G_data(4,8),G_data(4,10),G_data(4,7),G_data(4,12),G_data(4,14),G_data(4,5)]  Reactances2=[G_data(4,6),G_data(4,8),G_data(4,10),G_data(4,7),G_data(4,14),G_data(4,5)]  dAxisTimeConstants=Open-circuit  qAxisTimeConstants=Open-circuit  TimeConstants1="[G_data(4,9)  G_data(4,11)  G_data(4,15)]"  TimeConstants2="[G_data(4,9)  G_data(4,11)  G_data(4,13)  G_data(4,15)]"  TimeConstants3="[  5.9  0.033  0.023  ]"  TimeConstants4=[ 8.0, 0.03, 0.3371, 0.0295 ]  TimeConstants5=[ 1.01, 0.053, 0.1 ]  TimeConstants6=[ 1.3201, 0.023, 1.0, 0.07 ]  TimeConstants7="[  1.01  0.053  0.051266  ]"  TimeConstants8=[ 1.3201, 0.0231, 0.3371, 0.0295 ]  StatorResistance=0  Mechanical="[ G_data(4,4) 0  4 ]"  PolePairs=4  InitialConditions=[0 -19.7189 0.713768 0.713768 0.713768 11.8538 -108.146 131.854 2.17091]  SetSaturation=off  Saturation=[0.6404,0.7127,0.8441,0.9214,0.9956,1.082,1.19,1.316,1.457;0.7,0.7698,0.8872,0.9466,0.9969,1.046,1.1,1.151,1.201]  LoadFlowParameters=[1 1500000000 20000 0 0]  TsPowergui=0  TsBlock=-1  IterativeModel=Forward Euler  IterativeDiscreteModel=Trapezoidal non iterative  BusType=PV  Pref=p(4,3)*1e6  Qref=0  Qmin=-inf  Qmax=inf  PLF=0  QLF=0
      settings: SourceProductName=Simscape Power Systems
  AC4A Excitation System 203 : sps_avr/AC4A Excitation System  Tr=Exc(4,2)  KaTa="[Exc(4,3)   Exc(4,4)]"  VIminmax=[-10 10]  VRminmax=[-4.53 5.64]  TbTc="[Exc(4,5)  Exc(4,6)]"  Kc=0  v0=[1 2.1709]  TsBlock=0
      settings: SourceProductName=Simscape Power Systems  SourceProductBaseCode=PS
  Bus Selector1 : BusSelector  OutputSignals="Mechanical.Rotor speed  wm  (pu),Output active power   Peo (pu),Mechanical.Rotor speed deviation  dw (pu),Mechanical.Rotor angle deviation  d_theta (rad),Mechanical.Rotor mechanical angle  theta (deg),dq0 components.Stator voltage  vd (pu),dq0 components.Stator voltage  vq (pu),dq0 components.Field current  ifd (pu),Output reactive power  Qeo (pu)"
  Complex to Magnitude-Angle : ComplexToMagnitudeAngle  Output=Magnitude
  "Delta Pa PSS 203 " : powerlib/Machines/Generic Power System Stabilizer  Tsensor=15e-3  K=2.5*1.25  Twashout=1  Tleadlag1=[60e-3 1]  Tleadlag2=[0 0]  VSlimits=[-0.15 0.15]  Vinit=0  Plot_On=off  MagdB_On=on  FreqRange=logspace(-2,2,500)
      settings: SourceProductName=Simscape Power Systems  SourceProductBaseCode=PS
  "Delta w PSS (Kundur) 203 " : powerlib/Machines/Generic Power System Stabilizer  Tsensor=15e-3  K=30  Twashout=10  Tleadlag1=[50e-3 20e-3]  Tleadlag2=[3 5.4]  VSlimits=[-0.15 0.15]  Vinit=0  Plot_On=off  MagdB_On=on  FreqRange=logspace(-2,2,500)
      settings: SourceProductName=Simscape Power Systems  SourceProductBaseCode=PS
  "MB-PSS 203 " : powerlib/Machines/Multi-Band Power System Stabilizer  OperationMode=Simplified settings  Kg=G  GL="[FL  KL]"  GI="[FI  KI]"  GH="[FH  KH]"  GLd=[66 66 9.4]  TcLF=[1.667 2 0 0 0 0 2 2.4 0 0 0 0 1 1]  GId=[66 66 47.6]  TcIF=[1 1 0.25 0.3 0 0 1 1 0.3 0.36 0 0 0 0]  GHd=[66 66 233]  TcHF="[0.01 0.012 0 0 0 0  0.012 0.0144 0 0 0 0 1 1]"  LIM=[.075 .15 .15 .15]  Plot_On=off  MagdB_On=off  FreqRange=logspace(-2,2,500)
      settings: SourceProductName=Simscape Power Systems  SourceProductBaseCode=PS
  Multiport Switch1 : MultiPortSwitch  Inputs=4  InputSameDT=on
  PSS model3 : Constant  Value=0
  PSS model4 : Constant
  Pref1 : Constant  Value=0.67495
  Real-Imag to Complex : RealImagToComplex
  STG 203 : powerlib/Machines/Steam Turbine and Governor  gentype=Tandem-compound (single mass)  reg1="[ 1  0.05    0 ]"  reg2="[ 0.001  0.15 ]"  reg3="[ -0.1  0.1  0  4.496 ]"  N=3000  turb1="[ 0  10   3.3   0.5   ]"  turb2="[   0   0.36    0.36   0.28   ]"  HA="[ 0.046  1.430  1.465   0.192 ]"  KA="[ 90.44  53.88  64.59   62.94  ]"  DA="[ 0.0115  0.3575  0.3663   0.0137  ]"  ini1=0.67495  ini2=[0.779316,-31.4247]
      settings: SourceProductName=Simscape Power Systems  SourceProductBaseCode=PS
  Scope4 : Scope
  Sum2 : Sum  SaturateOnIntegerOverflow=on  InputSameDT=on  OutDataTypeStr=Inherit: Same as first input
  Sum3 : Sum  Inputs=-+  SaturateOnIntegerOverflow=on  InputSameDT=on  OutDataTypeStr=Inherit: Same as first input
  Terminator1 : Terminator
  Terminator2 : Terminator
  Terminator3 : Terminator
  Vref203 : Constant
  wref : Constant
  A : PMIOPort  Port=1  Side=Left
  B : PMIOPort  Port=2  Side=Left
  C : PMIOPort  Port=3  Side=Left
  tag scope: EFD203=global, Pa203=global, Pe203=global, Pm203=global, Q203=global, Vt203=global, d_theta203=global, pss203=global, theta203=global, w203=global
  wires:
  Bus Selector1/7 -> Real-Imag to Complex/2  "<Stator voltage  vq (pu)>"
  Bus Selector1/6 -> Real-Imag to Complex/1  "<Stator voltage  vd (pu)>"
  wref/1 -> STG 203/1
  Vref203/1 -> AC4A Excitation System 203/1
  Bus Selector1/4 -> STG 203/4, [d_theta203]  "<Rotor angle deviation  d_theta (rad)>"
  203/1 -> [M203], Bus Selector1/1
  Bus Selector1/1 -> [w203], STG 203/3  "<Rotor speed  wm  (pu)>"
  Bus Selector1/3 -> "Delta w PSS (Kundur) 203 "/1, "MB-PSS 203 "/1  "<Rotor speed deviation  dw (pu)>"
  Real-Imag to Complex/1 -> Complex to Magnitude-Angle/1
  Complex to Magnitude-Angle/1 -> AC4A Excitation System 203/2, [Vt203]
  AC4A Excitation System 203/1 -> 203/2, [EFD203]
  Bus Selector1/5 -> [theta203]  "<Rotor mechanical angle  theta (deg)>"
  Bus Selector1/2 -> [Pe203]  "<Output active power   Peo (pu)>"
  Bus Selector1/8 -> AC4A Excitation System 203/3  "<Field current  ifd (pu)>"
  STG 203/4 -> 203/1, [Pm203]
  Bus Selector1/9 -> [Q203]  "<Output reactive power  Qeo (pu)>"
  PSS model4/1 -> Sum2/2
  Sum2/1 -> Multiport Switch1/1
  [PSSmodel] -> Sum2/1
  PSS model3/1 -> Multiport Switch1/2
  Sum3/1 -> [Pa203], "Delta Pa PSS 203 "/1  "Pm-Pe"
  "Delta Pa PSS 203 "/1 -> Multiport Switch1/5
  "Delta w PSS (Kundur) 203 "/1 -> Multiport Switch1/4
  [Pm203] -> Sum3/2
  [Pe203] -> Sum3/1
  "MB-PSS 203 "/1 -> Multiport Switch1/3
  STG 203/1 -> Terminator3/1
  STG 203/2 -> Terminator1/1
  STG 203/3 -> Terminator2/1
  Pref1/1 -> STG 203/2
  Multiport Switch1/1 -> AC4A Excitation System 203/4, Scope4/1, [pss203]
  connections:
  203/RConn1 -- A/RConn1
  203/RConn2 -- B/RConn1
  203/RConn3 -- C/RConn1

== system Australian14gen_R2017a/YPS_3 ==
  302 : powerlib/Machines/Synchronous Machine pu Standard  PresetModel=No  MechanicalLoad=Mechanical power Pm  ShowDetailedParameters=on  RotorType=Salient-pole  Units=per unit standard parameters  MeasurementBus=off  NominalParameters="[G_data(7,2)*1E6  G_data(7,3)*1E3  50]"  Reactances1=[G_data(7,6),G_data(7,8),G_data(7,10),G_data(7,7),G_data(7,12),G_data(7,14),G_data(7,5)]  Reactances2=[G_data(7,6),G_data(7,8),G_data(7,10),G_data(7,7),G_data(7,14),G_data(7,5)]  dAxisTimeConstants=Open-circuit  qAxisTimeConstants=Open-circuit  TimeConstants1="[G_data(7,9)  G_data(7,11)  G_data(7,15)]"  TimeConstants2="[G_data(7,9)  G_data(7,11)  G_data(7,13)  G_data(7,15)]"  TimeConstants3="[  5.9  0.033  0.023  ]"  TimeConstants4=[ 8.0, 0.03, 0.3371, 0.0295 ]  TimeConstants5=[ 1.01, 0.053, 0.1 ]  TimeConstants6=[ 1.3201, 0.023, 1.0, 0.07 ]  TimeConstants7="[  1.01  0.053  0.051266  ]"  TimeConstants8=[ 1.3201, 0.0231, 0.3371, 0.0295 ]  StatorResistance=0  Mechanical="[ G_data(7,4) 0  4 ]"  PolePairs=4  InitialConditions=[0 -64.0096 0.72008 0.72008 0.72008 -30.8729 -150.873 89.1271 1.91163]  SetSaturation=off  Saturation=[0.6404,0.7127,0.8441,0.9214,0.9956,1.082,1.19,1.316,1.457;0.7,0.7698,0.8872,0.9466,0.9969,1.046,1.1,1.151,1.201]  LoadFlowParameters=[1 939900000 20000 0 0]  TsPowergui=0  TsBlock=-1  IterativeModel=Forward Euler  IterativeDiscreteModel=Trapezoidal non iterative  BusType=PV  Pref=p(7,3)*1e6  Qref=0  Qmin=-inf  Qmax=inf  PLF=0  QLF=0
      settings: SourceProductName=Simscape Power Systems
  AC1A Excitation System 302 : sps_avr/AC1A Excitation System  Tr=Exc(7,2)  KaTa="[Exc(7,3)   Exc(7,4)]"  VAminmax=[-14.5 14.5]  VRminmax=[-5.43 6.03]  KfTf="[Exc(7,9)  Exc(7,10)]"  TbTc="[Exc(7,5)  Exc(7,6)]"  KeTe="[Exc(7,7)  Exc(7,8)]"  Ve12=[4.18 3.14]  SeVe12=[0.10 0.03]  Kd=0.38  Kc=0.20  v0=[1 1.9116]  TsBlock=0
      settings: SourceProductName=Simscape Power Systems  SourceProductBaseCode=PS
  Bus Selector1 : BusSelector  OutputSignals="Mechanical.Rotor speed  wm  (pu),Output active power   Peo (pu),Mechanical.Rotor speed deviation  dw (pu),Mechanical.Rotor angle deviation  d_theta (rad),Mechanical.Rotor mechanical angle  theta (deg),dq0 components.Stator voltage  vd (pu),dq0 components.Stator voltage  vq (pu),dq0 components.Field current  ifd (pu),Output reactive power  Qeo (pu)"
  Complex to Magnitude-Angle : ComplexToMagnitudeAngle  Output=Magnitude
  Delta Pa PSS 302 : powerlib/Machines/Generic Power System Stabilizer  Tsensor=15e-3  K=2.5*1.25  Twashout=1  Tleadlag1=[60e-3 1]  Tleadlag2=[0 0]  VSlimits=[-0.15 0.15]  Vinit=0  Plot_On=off  MagdB_On=on  FreqRange=logspace(-2,2,500)
      settings: SourceProductName=Simscape Power Systems  SourceProductBaseCode=PS
  Delta w PSS (Kundur) 302 : powerlib/Machines/Generic Power System Stabilizer  Tsensor=15e-3  K=30  Twashout=10  Tleadlag1=[50e-3 20e-3]  Tleadlag2=[3 5.4]  VSlimits=[-0.15 0.15]  Vinit=0  Plot_On=off  MagdB_On=on  FreqRange=logspace(-2,2,500)
      settings: SourceProductName=Simscape Power Systems  SourceProductBaseCode=PS
  "MB-PSS 302 " : powerlib/Machines/Multi-Band Power System Stabilizer  OperationMode=Simplified settings  Kg=G  GL="[FL  KL]"  GI="[FI  KI]"  GH="[FH  KH]"  GLd=[66 66 9.4]  TcLF=[1.667 2 0 0 0 0 2 2.4 0 0 0 0 1 1]  GId=[66 66 47.6]  TcIF=[1 1 0.25 0.3 0 0 1 1 0.3 0.36 0 0 0 0]  GHd=[66 66 233]  TcHF="[0.01 0.012 0 0 0 0  0.012 0.0144 0 0 0 0 1 1]"  LIM=[.075 .15 .15 .15]  Plot_On=off  MagdB_On=off  FreqRange=logspace(-2,2,500)
      settings: SourceProductName=Simscape Power Systems  SourceProductBaseCode=PS
  Multiport Switch1 : MultiPortSwitch  Inputs=4  InputSameDT=on
  PSS model3 : Constant  Value=0
  PSS model4 : Constant
  Pref1 : Constant  Value=0.705
  Real-Imag to Complex : RealImagToComplex
  STG 302 : powerlib/Machines/Steam Turbine and Governor  gentype=Tandem-compound (single mass)  reg1="[ 1  0.05    0 ]"  reg2="[ 0.001  0.15 ]"  reg3="[ -0.1  0.1  0  4.496 ]"  N=3000  turb1="[ 0  10   3.3   0.5   ]"  turb2="[   0   0.36    0.36   0.28   ]"  HA="[ 0.046  1.430  1.465   0.192 ]"  KA="[ 90.44  53.88  64.59   62.94  ]"  DA="[ 0.0115  0.3575  0.3663   0.0137  ]"  ini1=0.705  ini2=[0.779316,-31.4247]
      settings: SourceProductName=Simscape Power Systems  SourceProductBaseCode=PS
  Scope4 : Scope
  Sum2 : Sum  SaturateOnIntegerOverflow=on  InputSameDT=on  OutDataTypeStr=Inherit: Same as first input
  Sum3 : Sum  Inputs=-+  SaturateOnIntegerOverflow=on  InputSameDT=on  OutDataTypeStr=Inherit: Same as first input
  Terminator1 : Terminator
  Terminator2 : Terminator
  Terminator3 : Terminator
  Vref302 : Constant
  wref : Constant
  A : PMIOPort  Port=1  Side=Left
  B : PMIOPort  Port=2  Side=Left
  C : PMIOPort  Port=3  Side=Left
  tag scope: EFD302=global, Pa302=global, Pe302=global, Pm302=global, Q302=global, Vt302=global, d_theta302=global, pss302=global, theta302=global, w302=global
  wires:
  Bus Selector1/7 -> Real-Imag to Complex/2  "<Stator voltage  vq (pu)>"
  Bus Selector1/6 -> Real-Imag to Complex/1  "<Stator voltage  vd (pu)>"
  wref/1 -> STG 302/1
  Vref302/1 -> AC1A Excitation System 302/1
  Bus Selector1/4 -> STG 302/4, [d_theta302]  "<Rotor angle deviation  d_theta (rad)>"
  302/1 -> Bus Selector1/1, [M302]
  Bus Selector1/1 -> [w302], STG 302/3  "<Rotor speed  wm  (pu)>"
  Bus Selector1/3 -> Delta w PSS (Kundur) 302/1, "MB-PSS 302 "/1  "<Rotor speed deviation  dw (pu)>"
  Real-Imag to Complex/1 -> Complex to Magnitude-Angle/1
  Complex to Magnitude-Angle/1 -> AC1A Excitation System 302/2, [Vt302]
  AC1A Excitation System 302/1 -> 302/2, [EFD302]
  Bus Selector1/5 -> [theta302]  "<Rotor mechanical angle  theta (deg)>"
  Bus Selector1/2 -> [Pe302]  "<Output active power   Peo (pu)>"
  Bus Selector1/8 -> AC1A Excitation System 302/3  "<Field current  ifd (pu)>"
  STG 302/4 -> 302/1, [Pm302]
  Bus Selector1/9 -> [Q302]  "<Output reactive power  Qeo (pu)>"
  PSS model4/1 -> Sum2/2
  Sum2/1 -> Multiport Switch1/1
  [PSSmodel] -> Sum2/1
  PSS model3/1 -> Multiport Switch1/2
  Sum3/1 -> [Pa302], Delta Pa PSS 302/1  "Pm-Pe"
  Delta Pa PSS 302/1 -> Multiport Switch1/5
  Delta w PSS (Kundur) 302/1 -> Multiport Switch1/4
  [Pm302] -> Sum3/2
  [Pe302] -> Sum3/1
  "MB-PSS 302 "/1 -> Multiport Switch1/3
  STG 302/1 -> Terminator3/1
  STG 302/2 -> Terminator1/1
  STG 302/3 -> Terminator2/1
  Pref1/1 -> STG 302/2
  Multiport Switch1/1 -> AC1A Excitation System 302/4, Scope4/1, [pss302]
  connections:
  302/RConn1 -- A/RConn1
  302/RConn2 -- B/RConn1
  302/RConn3 -- C/RConn1
